simulink library "Power_Shaft2_Electric_A1_A2"  (R2026a)
settings: Solver=VariableStepAuto
undefined symbols (not defined in the file): Powertrain, ShaftA1, ShaftA2
libraries: Power_Components x3, fl_lib x2, sm_lib x1, Cooling_Motor2 x1
Description:
  | Component of Simscape Vehicle Templates Library
  | 
  | Copyright 2018-2026 The MathWorks, Inc.
settings Model: Creator=smiller  LastModifiedBy=smiller

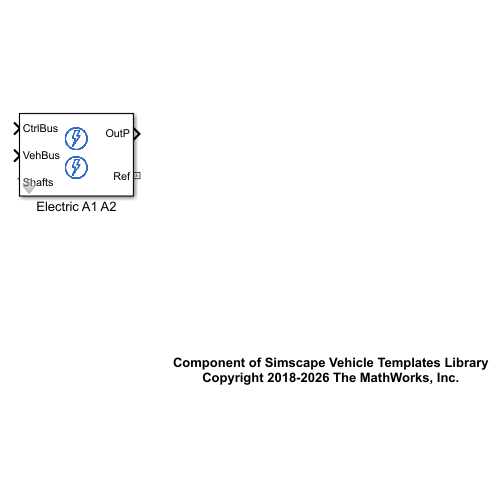
[thumbnail: Simulink's stored preview of the top-level diagram]
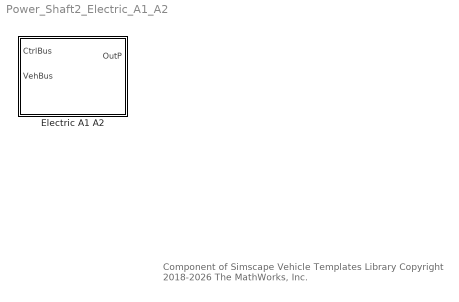
== system Power_Shaft2_Electric_A1_A2 ==
  note: Component of Simscape Vehicle Templates Library
      | Copyright 2018-2026 The MathWorks, Inc.
  Electric A1 A2 : Subsystem  VariantControl=ElectricTwoMotor  mask(Electric Propulsion with Two Motors){Power=Powertrain.Power, InitTriggerDropdown=0}
      mask prompts: Power "Power 2 Motor (Structure)"; InitTriggerDropdown "Initialization Trigger Dropdown"
      mask help: Two electric motors with optional cooling system. Physical connections for the motor shafts are in bus Shafts.
      mask init:
      | curblk = gcb;
      | 
      | % Trigger Mask Initialization for 
      | % variant subsystems below this level
      | sm_car_lib_maskInitTrigger(curblk)
      mask TypeOptions InitTriggerDropdown: 0 | 1
      mask Display: image('sm_car_vehicle_power_e2motor_IMAGE.png');

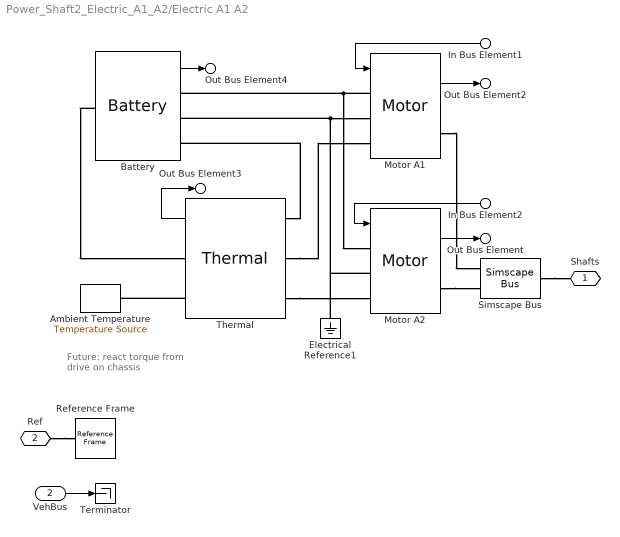
== system Power_Shaft2_Electric_A1_A2/Electric A1 A2 ==
  note: Future:
      | react torque
      | from drive
      | on chassis
  In Bus Element1 : Inport  PortName=CtrlBus  Element=MMotorA1Demand
  In Bus Element2 : Inport  PortName=CtrlBus  Element=MMotorA2Demand
  VehBus : Inport  Port=2
  Ambient Temperature : fl_lib/Thermal/Thermal Sources/Temperature Source  temperature=Power.TAmbient.Value K
  Battery : Power_Components/Battery  SystemSampleTime=-1  VariantActivationTime=update diagram  EmptyChoice=off  PassThrough=off  PassThroughVariantControl=(default)  EmptyChoiceVariantControl=(default)  AllowFlexibleInterface=on  Latency=0  AutoFrameSizeCalculation=off
  Electrical Reference1 : fl_lib/Electrical/Electrical Elements/Electrical Reference
  Motor A1 : Power_Components/Motor  Motor=Power.MotorA1
  Motor A2 : Power_Components/Motor  Motor=Power.MotorA2
  Reference Frame : sm_lib/Frames and Transforms/Reference Frame
  Simscape Bus : SimscapeBus  HierarchyStrings=ShaftA1;ShaftA2
  Terminator : Terminator
  Thermal : Cooling_Motor2/Thermal  VariantControl=Variant1  VariantLabel=Power.Cooling.class.Value  InitTriggerDropdown=0
      settings: AttributesFormatString=%<ActiveVariant>
  Shafts : PMIOPort  Side=Left
  Ref : PMIOPort  Port=2  Side=Right
  Out Bus Element : Outport  VectorParamsAs1DForOutWhenUnconnected=off  PortName=OutP  Element=MotorA2
  Out Bus Element2 : Outport  VectorParamsAs1DForOutWhenUnconnected=off  PortName=OutP  Element=MotorA1
  Out Bus Element3 : Outport  VectorParamsAs1DForOutWhenUnconnected=off  PortName=OutP  Element=Thermal
  Out Bus Element4 : Outport  VectorParamsAs1DForOutWhenUnconnected=off  PortName=OutP  Element=Battery
  wires:
  Motor A2/1 -> Out Bus Element/1
  In Bus Element2/1 -> Motor A2/1
  In Bus Element1/1 -> Motor A1/1
  Motor A1/1 -> Out Bus Element2/1
  Thermal/1 -> Out Bus Element3/1
  VehBus/1 -> Terminator/1
  Battery/1 -> Out Bus Element4/1
  connections:
  Motor A1/LConn1 -- Battery/RConn1 -- Motor A2/LConn1
  Motor A2/LConn2 -- Electrical Reference1/LConn1 -- Battery/RConn2 -- Motor A1/LConn2
  Motor A1/RConn1 -- Simscape Bus/LConn1
  Simscape Bus/RConn1 -- Shafts/RConn1
  Ref/RConn1 -- Reference Frame/RConn1
  Motor A2/RConn1 -- Simscape Bus/LConn2
  Thermal/LConn1 -- Battery/RConn3
  Thermal/LConn2 -- Motor A1/LConn3
  Thermal/LConn3 -- Motor A2/LConn3
  Thermal/RConn2 -- Ambient Temperature/LConn1
  Battery/LConn1 -- Thermal/RConn1
